simulink model "heater_on_off_2023b"  (R2023b)
settings: Solver=VariableStepAuto  StartTime=0.0  StopTime=40.0  RelTol=1e-3
values from neighbouring files (symbols this model uses):
  C = 10    [heater_params.m]
  k = 1    [heater_params.m]
  q = 200    [heater_params.m]
  T0 = 0    [heater_params.m]
  Te = 10    [heater_params.m]
  Tref = 100    [heater_params.m]
settings Model: Creator=martinhaugen  LastModifiedBy=martinhaugen
settings RTWCC: GPUComputeCapability=5.0

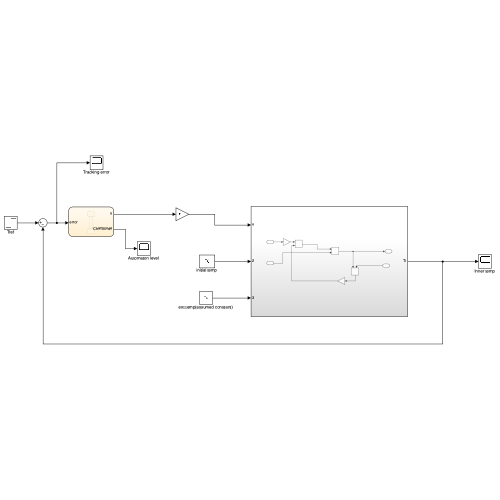
[thumbnail: Simulink's stored preview of the top-level diagram]
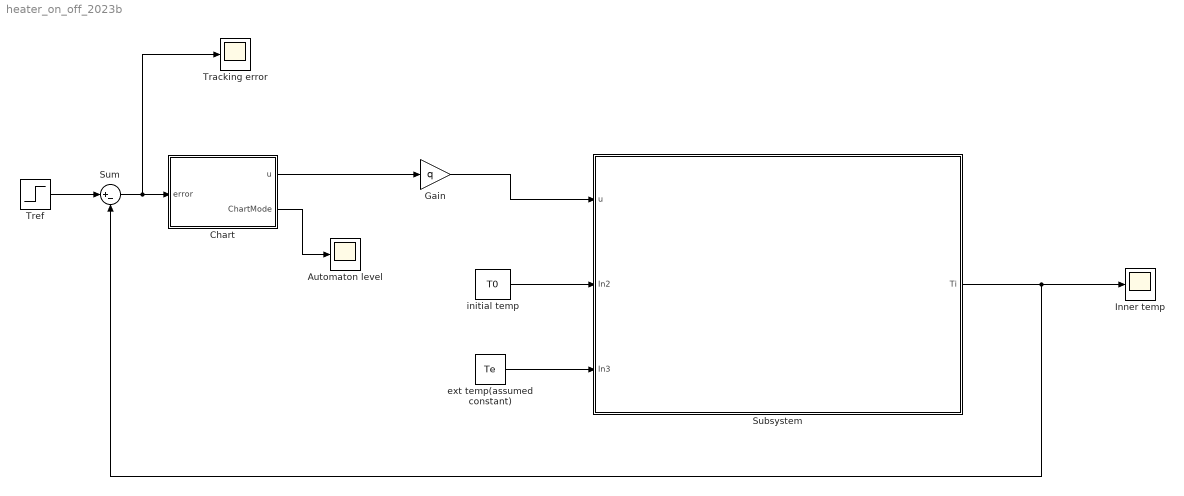
== system heater_on_off_2023b ==
  Automaton level : Scope
  Chart : Stateflow chart  TreatAsAtomicUnit=on
  Gain : Gain  Gain=q
  Inner temp : Scope
  Subsystem : Subsystem
  Sum : Sum  Inputs=|+-
  Tracking error : Scope
  Tref : Step  Time=0  After=Tref  SampleTime=0
  ext temp(assumed constant) : Constant  Value=Te
  initial temp : Constant  Value=T0
  wires:
  Chart/1(u) -> Gain/1
  initial temp/1 -> Subsystem/2(In2)
  ext temp(assumed constant)/1 -> Subsystem/3(In3)
  Subsystem/1(Ti) -> Sum/2, Inner temp/1
  Tref/1 -> Sum/1
  Sum/1 -> Tracking error/1, Chart/1(error)
  Chart/2(ChartMode) -> Automaton level/1
  Gain/1 -> Subsystem/1(u)

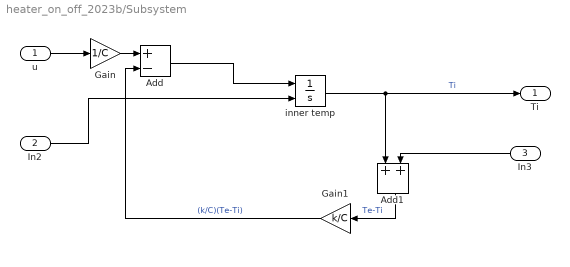
== system heater_on_off_2023b/Subsystem ==
  u : Inport
  In2 : Inport  Port=2
  In3 : Inport  Port=3
  Add : Sum  Inputs=+-
  Add1 : Sum
  Gain : Gain  Gain=1/C
  Gain1 : Gain  Gain=k/C
  inner temp : Integrator  InitialConditionSource=external
  Ti : Outport
  wires:
  In3/1 -> Add1/2
  In2/1 -> inner temp/2
  Gain/1 -> Add/1
  u/1 -> Gain/1
  inner temp/1 -> Ti/1, Add1/1  "Ti"
  Add/1 -> inner temp/1
  Gain1/1 -> Add/2  "(k/C)(Te-Ti)"
  Add1/1 -> Gain1/1  "Te-Ti"

== stateflow chart heater_on_off_2023b/Chart ==
  settings: updateMethod=CONTINUOUS
  state HEATING
    entry:
    u=1;
  state COOLING
    entry:
    u=0;
  (default) -> HEATING
  COOLING -> HEATING : [error >= epsilon]
  HEATING -> COOLING : [error <= -epsilon]
  data: epsilon parameter; u output; error input; ChartMode output Enum: ChartModeType
